simulink model "sanityCheck"  (R2018a)
settings: Solver=VariableStepAuto  StartTime=0.0  StopTime=500  RelTol=1e-3
values from neighbouring files (symbols this model uses):
  bb = 0.254    [RLDesignJoystick.m]
  I = 0.762    [RLDesignJoystick.m]
undefined symbols (not defined in the file or in its folder): a2, b2, K2, U
libraries: simulink x1
settings Model: Creator=travis  LastModifiedBy=transmogrifier

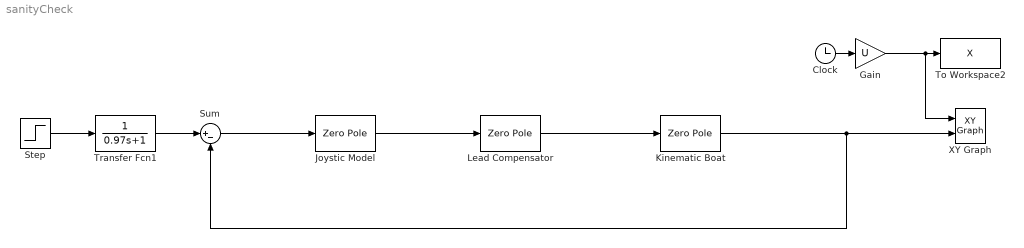
== system sanityCheck ==
  Clock : Clock
  Gain : Gain  Gain=U
  Joystic Model : ZeroPole  Zeros=[]  Poles=[0 -bb/I]  Gain=[I]
  Kinematic Boat : ZeroPole  Zeros=[]  Poles=[0 0 -5/4]  Gain=[U/100]
  Lead Compensator : ZeroPole  Zeros=[-b2]  Poles=[-a2]  Gain=[K2]
  Step : Step  Time=10  SampleTime=0
  Sum : Sum  Inputs=|+-
  To Workspace2 : ToWorkspace  VariableName=X  SaveFormat=Timeseries  SampleTime=-1
  Transfer Fcn1 : TransferFcn  Denominator=[0.97 1]
  XY Graph : simulink/Sinks/XY Graph  xmin=-10  xmax=U*500  ymin=-20  ymax=20  st=-1
  wires:
  Lead Compensator/1 -> Kinematic Boat/1
  Sum/1 -> Joystic Model/1
  Clock/1 -> Gain/1
  Gain/1 -> XY Graph/1, To Workspace2/1
  Kinematic Boat/1 -> Sum/2, XY Graph/2
  Step/1 -> Transfer Fcn1/1
  Joystic Model/1 -> Lead Compensator/1
  Transfer Fcn1/1 -> Sum/1
